simulink model "lab6_Den"  (R2017b)
settings: Solver=VariableStepAuto  StartTime=0.0  StopTime=50  FixedStep=0.001  MaxStep=0.001  RelTol=1e-4
settings Model: Creator=user  LastModifiedBy=anton
settings SolverCC: AutoInsertRateTranBlk=on
settings DataIOCC: LimitDataPoints=on  SaveOutput=off  SignalLogging=off  SaveTime=off
settings OptimizationCC: LifeSpan=inf
settings DebuggingCC: AlgebraicLoopMsg=error  SingleTaskRateTransMsg=error  AllowSymbolicDim=off  SFUnexpectedBacktrackingDiag=warning  SFNoUnconditionalDefaultTransitionDiag=warning  SFExecutionAtInitializationDiag=none
settings CodeAppCC: StateflowObjectComments=on
settings GRTTargetCC: TargetLangStandard=C89/C90 (ANSI)  GeneratePreprocessorConditionals=Disable all
settings ConfigComp: CovMetricSettings=dw  CovHtmlReporting=on  CovSaveCumulativeToWorkspaceVar=on  CovSaveSingleToWorkspaceVar=on  CovExternalEMLEnable=off

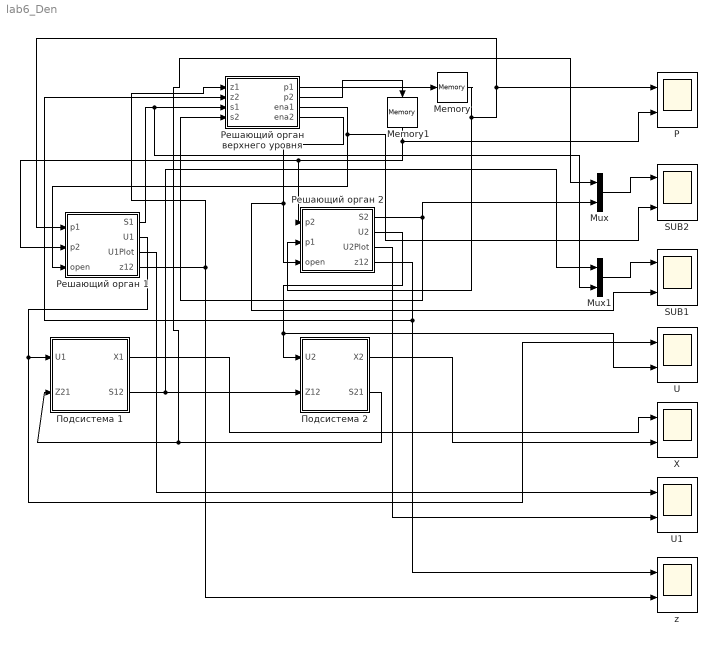
== system lab6_Den ==
  Memory : Memory
  Memory1 : Memory
  Mux : Mux  Inputs=2
  Mux1 : Mux  Inputs=2
  P : Scope  NumInputPorts=2
  SUB1 : Scope  NumInputPorts=2
  SUB2 : Scope  NumInputPorts=2
  U : Scope  NumInputPorts=2
  U1 : Scope  NumInputPorts=2
  X : Scope  NumInputPorts=2
  z : Scope  NumInputPorts=2
  Подсистема 1 : Subsystem
  Подсистема 2 : Subsystem
  Решающий орган 1 : Subsystem
  Решающий орган 2 : Subsystem
  Решающий орган верхнего уровня : MATLAB Function  TreatAsAtomicUnit=on
  wires:
  Подсистема 1/2(S12) -> Mux1/1, Подсистема 2/2(Z12)
  Подсистема 2/2(S21) -> Mux/1, Подсистема 1/2(Z21)
  Подсистема 1/1(X1) -> X/1
  Подсистема 2/1(X2) -> X/2
  Решающий орган верхнего уровня/1(p1) -> Memory/1
  Решающий орган верхнего уровня/2(p2) -> Memory1/1
  Memory/1 -> Решающий орган 2/2(p1), Решающий орган 1/1(p1), P/1
  Memory1/1 -> Решающий орган 2/1(p2), Решающий орган 1/2(p2), P/2
  Решающий орган 1/1(S1) -> Mux1/2, Решающий орган верхнего уровня/3(s1)
  Решающий орган 2/1(S2) -> Mux/2, Решающий орган верхнего уровня/4(s2)
  Решающий орган 1/2(U1) -> Подсистема 1/1(U1), U/1
  Решающий орган 2/2(U2) -> Подсистема 2/1(U2), U/2
  Решающий орган верхнего уровня/3(ena1) -> SUB2/2, Решающий орган 1/3(open)
  Решающий орган верхнего уровня/4(ena2) -> SUB1/2, Решающий орган 2/3(open)
  Mux/1 -> SUB2/1
  Mux1/1 -> SUB1/1
  Решающий орган 1/3(U1Plot) -> U1/1
  Решающий орган 2/3(U2Plot) -> U1/2
  Решающий орган 2/4(z12) -> Решающий орган верхнего уровня/2(z2), z/1
  Решающий орган 1/4("z12 ") -> Решающий орган верхнего уровня/1(z1), z/2

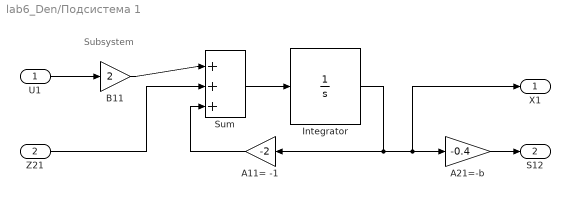
== system lab6_Den/Подсистема 1 ==
  note: Subsystem
  U1 : Inport
  Z21 : Inport  Port=2
  A11= -1 : Gain  Gain=-2
  A21=-b : Gain  Gain=-0.4
  B11 : Gain  Gain=2
  Integrator : Integrator
  Sum : Sum  Inputs=|+++
  X1 : Outport
  S12 : Outport  Port=2
  wires:
  U1/1 -> B11/1
  Integrator/1 -> A21=-b/1, X1/1, A11= -1/1
  A11= -1/1 -> Sum/3
  Sum/1 -> Integrator/1
  Z21/1 -> Sum/2
  A21=-b/1 -> S12/1
  B11/1 -> Sum/1

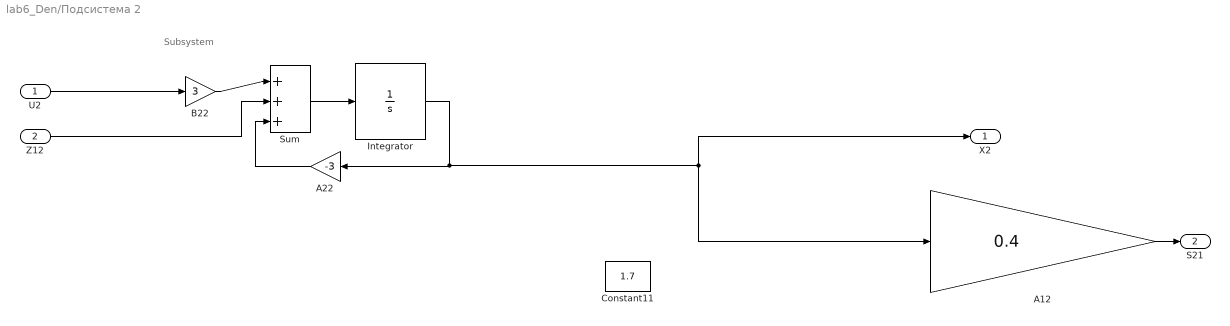
== system lab6_Den/Подсистема 2 ==
  note: Subsystem
  U2 : Inport
  Z12 : Inport  Port=2
  A12 : Gain  Gain=0.4
  A22 : Gain  Gain=-3
  B22 : Gain  Gain=3
  Constant11 : Constant  Value=1.7
  Integrator : Integrator
  Sum : Sum  Inputs=|+++
  X2 : Outport
  S21 : Outport  Port=2
  wires:
  U2/1 -> B22/1
  A12/1 -> S21/1
  Z12/1 -> Sum/2
  Integrator/1 -> A12/1, X2/1, A22/1
  A22/1 -> Sum/3
  Sum/1 -> Integrator/1
  B22/1 -> Sum/1

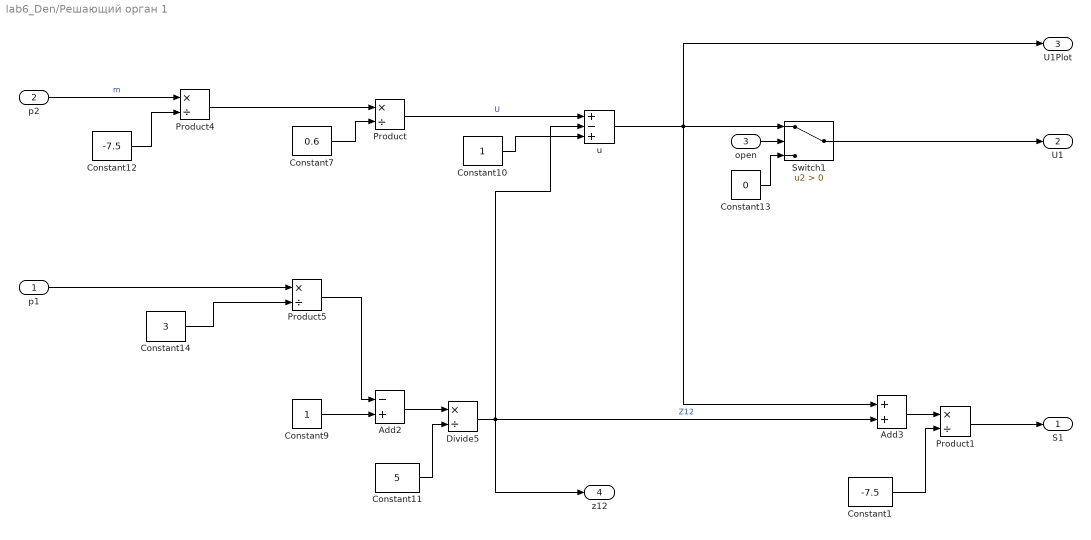
== system lab6_Den/Решающий орган 1 ==
  p1 : Inport
  p2 : Inport  Port=2
  open : Inport  Port=3
  Add2 : Sum  Inputs=-+
  Add3 : Sum
  Constant1 : Constant  Value=-7.5
  Constant10 : Constant
  Constant11 : Constant  Value=5
  Constant12 : Constant  Value=-7.5
  Constant13 : Constant  Value=0
  Constant14 : Constant  Value=3
  Constant7 : Constant  Value=0.6
  Constant9 : Constant
  Divide5 : Product  Inputs=*/
  Product{,1,4..5} (4 alike) : Product  Inputs=*/
  Switch1 : Switch  Criteria=u2 > Threshold
  u : Sum  Inputs=+-+
  S1 : Outport
  U1 : Outport  Port=2
  U1Plot : Outport  Port=3
  "z12 " : Outport  Port=4
  wires:
  Switch1/1 -> U1/1
  Constant14/1 -> Product5/2
  Product4/1 -> Product/1
  Constant10/1 -> u/3
  Constant12/1 -> Product4/2
  u/1 -> U1Plot/1, Add3/1, Switch1/1
  p1/1 -> Product5/1
  open/1 -> Switch1/2
  p2/1 -> Product4/1  "m"
  Constant7/1 -> Product/2
  Add2/1 -> Divide5/1
  Product/1 -> u/1  "U"
  Product5/1 -> Add2/1
  Divide5/1 -> "z12 "/1, Add3/2, u/2  "Z12"
  Constant11/1 -> Divide5/2
  Constant9/1 -> Add2/2
  Constant13/1 -> Switch1/3
  Constant1/1 -> Product1/2
  Add3/1 -> Product1/1
  Product1/1 -> S1/1

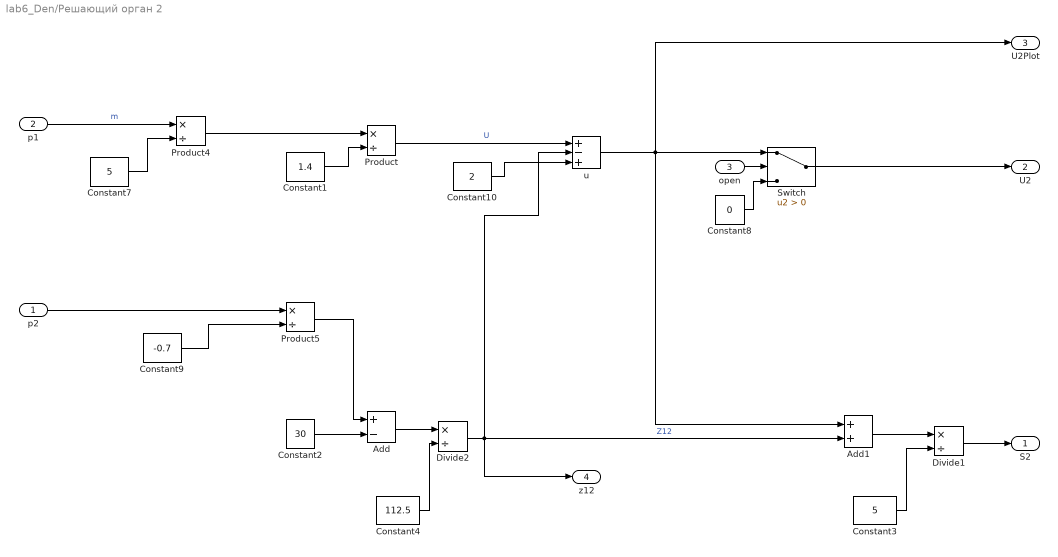
== system lab6_Den/Решающий орган 2 ==
  p2 : Inport
  p1 : Inport  Port=2
  open : Inport  Port=3
  Add : Sum  Inputs=+-
  Add1 : Sum
  Constant1 : Constant  Value=1.4
  Constant10 : Constant  Value=2
  Constant2 : Constant  Value=30
  Constant3 : Constant  Value=5
  Constant4 : Constant  Value=112.5
  Constant7 : Constant  Value=5
  Constant8 : Constant  Value=0
  Constant9 : Constant  Value=-0.7
  Divide1 : Product  Inputs=*/
  Divide2 : Product  Inputs=*/
  Product : Product  Inputs=*/
  Product4 : Product  Inputs=*/
  Product5 : Product  Inputs=*/
  Switch : Switch  Criteria=u2 > Threshold
  u : Sum  Inputs=+-+
  S2 : Outport
  U2 : Outport  Port=2
  U2Plot : Outport  Port=3
  z12 : Outport  Port=4
  wires:
  Constant2/1 -> Add/2
  Add/1 -> Divide2/1
  Constant4/1 -> Divide2/2
  p2/1 -> Product5/1
  Product/1 -> u/1  "U"
  Constant1/1 -> Product/2
  u/1 -> U2Plot/1, Add1/1, Switch/1
  Divide2/1 -> z12/1, Add1/2, u/2  "Z12"
  Switch/1 -> U2/1
  open/1 -> Switch/2
  Constant8/1 -> Switch/3
  p1/1 -> Product4/1  "m"
  Product4/1 -> Product/1
  Product5/1 -> Add/1
  Constant7/1 -> Product4/2
  Constant9/1 -> Product5/2
  Constant10/1 -> u/3
  Constant3/1 -> Divide1/2
  Divide1/1 -> S2/1
  Add1/1 -> Divide1/1

== matlab function lab6_Den/Решающий орган верхнего уровня ==
  settings: updateMethod=DISCRETE
  data: z1 input; p1 output; z2 input; s1 input; s2 input; p2 output; ena1 output; ena2 output
function [p1, p2, ena1, ena2] = fcn(z1, z2, s1, s2)
persistent p1_t;
persistent p2_t;
persistent ena1_t;
persistent ena2_t;
eps =  0.005;  % Величина отклонения оценки от реального значения
step = 0.0025;  % Шаг изменения множителей p
% Инициализация
if(isempty(p1_t))
    p1_t =-1.0;%4;%-5;% 1.5;
    p2_t =-1;%-4.0;%5;%-5;% -1.5;
    ena1_t = 0;%0
    ena2_t = 0;%0
    p1 = p1_t;
    p2 = p2_t;
    ena1 = ena1_t;
    ena2 = ena2_t;
    return;
end
% Коррекция множителя p1
if(abs(p2_t*z2-p2_t*s1+p1_t*z1-p1_t*s2) > eps)%(2*abs((p2_t*z2-p1_t*s1+p1_t*z1-p2_t*s2)/(abs(p1_t)+abs(p2_t))) > eps)%(abs((z1-s2)) > eps || abs((z2-s1)) > eps)
   % Знак перед step завистит от знака s2
   %p1_t = p1_t+step*(z1-(0.2)*s2);
   p1_t = p1_t+step*(z1-s2);
   ena1_t = 0; 
   
   %p2_t = p2_t+step*(z2-(-2/15)*s1);
   p2_t = p2_t+step*(z2-s1);
   ena2_t = 0; 
else
   ena1_t = 1;   
   ena2_t = 1; 
end
p1 = p1_t;
p2 = p2_t;
ena1 = ena1_t;
ena2 = ena2_t;
end
